simulink model "Nanogrid"  (R2026a)
settings: Solver=VariableStepAuto  StopTime=3
PreLoadFcn:
  | NanogridParam
undefined symbols (not defined in the file): baseLoad, bessSystem, bessVoltage, DiscIntNeverNeededParam, ee_sli_rtmsupport, gcbh, gflInverter, gfmInverter, nanoLoad, PV, PVInverter, ref, solar, solarInsolationChange, Ts
libraries: nesl_utility x51, eeGeneralControl x38, ee_lib x33, fl_lib x24, simulink x20, eeTransforms x13, slpidlib x8, nesl_utility_internal x4, sl_signal_attributes x4, sl_discontinuities x4, eeSinusoidalMeasurementV2 x3, batteryecm_lib x2
(part 2 of 6)

== system Nanogrid/BESS Integrated/Detailed/BESS Controller ==
  VRef : Inport
  FRef : Inport  Port=2
  PRef : Inport  Port=3
  QRef : Inport  Port=4
  Mode : Inport  Port=5
  Reset : Inport  Port=6
  VIBus : Inport  Port=7
  Grid Following : Subsystem  VariantControl=Grid Following  mask(Grid Following Controller){mp=gflInverter.activeDroop, mv=gflInverter.reactiveDroop, P=Real power, MVA=gflInverter.ratedPower, frequency=frequency, zbase=gflInverter.baseImpedance, L=filterInductance%gflInverter.filterInductance, Imax=gflInverter.iMaxPU, Td=gflInverter.sensorDelay, Kpic=gflInverter.kpId, Kiic=gflInverter.kiId, Kd=0}
      mask prompts: mp "Real power droop cofficient"; mv "Reactive power droop cofficient"; P "Priority mode"; MVA "Base Power (V*A)"; frequency "Frequency (Hz)"; zbase "Base Impedance (Ohm)"; L "Filter Inductance (H)"; Imax "Inverter current limit (pu)"; Td "Sensor time delay (s)"; Kpic "Proportional gain"; Kiic "Integral gain"; Kd "Derevative gain"
      mask help: This block implements a Grid Following control strategy where the BESS synchronizes with an existing grid voltage and frequency. Ideal for systems where the grid is strong and the BESS acts as a power source following grid conditions.
      settings: CopyFcn=set_param(gcb,'LinkStatus','none');
      mask TypeOptions P: Real power  | Reactive power
      mask DialogControl Container4 Prompt: General
      mask DialogControl Container5 Prompt: Current Controller
      mask Display: image('gridfollowing2_2_9_7_2_1_1.png');
  Grid Forming : Subsystem  VariantControl=Grid Forming  mask(Grid Forming Controller){power=plantRating*1000, girdLineVoltage=Vac, powerFreq=frequency, dcBusVoltage=bessVoltage, measSampleTime=gfmInverter.measurementSampleTime, powerControl=Virtual Synchronous Machine, activePowerSampleTime=gfmInverter.droopControl.sampleTime, droopSlope=gfmInverter.droopControl.freqSlopeMp*350, droopT1=gfmInverter.droopControl.T1, droopT2=gfmInverter.droopControl.T2, droopTC=gfmInverter.droopControl.lpfTimeConst, vsmPmeasFilterTC=gfmInverter.vsm.PmeasTimeConst, vsmFreqDroop=gfmInverter.vsm.freqDroop, vsmInertiaTC=gfmInverter.vsm.inertiaConstant, vsmDampingConst=gfmInverter.vsm.dampingCoefficent, dampingPowerMaxLimit=gfmInverter.vsm.maxDampingPower, dampingPowerMinLimit=gfmInverter.vsm.minDampingPower, freqMeasTimeConst=gfmInverter.freqMeasTimeConst, freqOption=Constant Frequency Reference, voltreference=gfmInverter.Qcontrol.voltageReference, QVoltFilterTC=gfmInverter.Qcontrol.QmeasTimeConst, QVoltDroop=gfmInverter.Qcontrol.voltageDroop, currentLimit=Current Limiting, maxSatCurrentLimit=1%gfmInverter.currentLimit.maxSaturationCurrent, maxVICurrentLimit=gfmInverter.currentLimit.viCurrentLimit, ctLimitVirtualImp=gfmInverter.currentLimit.virImpResistanceCoeff, ctLimitXbyR=gfmInverter.currentLimit.virImpXbyR, ctLimitDelayTime=gfmInverter.currentLimit.maxSaturationDelay, currentSatTime=gfmInverter.currentLimit.satCurrentRunTime, currentVITimeConst=gfmInverter.currentLimit.viFilterTimeConst, voltControlTs=gfmInverter.controller.VoltageControlSampleTime, vdPGain=gfmInverter.controller.voltControllerKp, VdIGain=gfmInverter.controller.voltControllerKi, VdMaxCt=gfmInverter.controller.voltageMaxId, VdMinCt=gfmInverter.controller.voltageMinId, VqPGain=gfmInverter.controller.voltControllerKp, VqIGain=gfmInverter.controller.voltControllerKi, VqMaxCt=gfmInverter.controller.voltageMaxIq, VqMinCt=gfmInverter.controller.voltageMinIq, vdvqLPFTimeConst=gfmInverter.controller.voltMeasTimeConst, currentControlTs=gfmInverter.controller.CurrentControlSampleTime, filterInductance=gfmInverter.L, IdPGain=gfmInverter.controller.ctControllerKp, IdIGain=gfmInverter.controller.ctControllerKi, IqPGain=gfmInverter.controller.ctControllerKp, IqIGain=gfmInverter.controller.ctControllerKi}
      mask prompts: power "Grid forming converter power (VA)"; girdLineVoltage "Grid line voltage (V)"; powerFreq "Grid frequency (Hz)"; dcBusVoltage "DC bus voltage"; measSampleTime "Measurement sample time"; powerControl "Active Power Control"; activePowerSampleTime "Sample time (s)"; droopSlope "Power droop slope (pu, Hz/W)"; droopT1 "Lead-Lag numerator time constant (s)"; droopT2 "Lead-Lag denominator time constant (s)"; droopTC "Filter cut-off time constant (s)"; vsmPmeasFilterTC "Power measurement filter time constant (s)"; vsmFreqDroop "Frequency droop (pu,  W/Hz)"; vsmInertiaTC "Inertia constant M (pu)"; vsmDampingConst "Damping constant (pu/Hz)"; dampingPowerMaxLimit "Damping power maximum limit (pu)"; dampingPowerMinLimit "Damping power minimum limit (pu)"; freqMeasTimeConst "Frequency measurement time constant (s)"; freqOption "Damping power fequency option"; voltreference "Voltage reference value (pu)"; QVoltFilterTC "Power measurement filter time constant (s)"; QVoltDroop "Voltage droop (pu, V/VAR)"; currentLimit "Current limiting method"; maxSatCurrentLimit "Maximum current saturation (pu)"; maxVICurrentLimit "Maximum virtual impedance current (pu)"; ctLimitVirtualImp "Virtual impedance coefficient (pu.Ohm/pu.A)"; ctLimitXbyR "Virtual X/R ratio"; ctLimitDelayTime "Maximum current delay time (s)"; currentSatTime "Current limiting run time (s)"; currentVITimeConst "Filter time constant (s)"; voltControlTs "Controller sample time (s)"; vdPGain "Vd proportional gain"; VdIGain "Vd integral gain"; VdMaxCt "Vd maximum current limit (A)"; VdMinCt "Vd minimum current limit (A)"; VqPGain "Vq proportional gain"; VqIGain "Vq integral gain"; VqMaxCt "Vq maximum current limit (A)"; VqMinCt "Vq minimum current limit (A)"; vdvqLPFTimeConst "Voltage measurement filter time constant (s)"; currentControlTs "Controller sample time (s)"; filterInductance "Filter inductance (H)"; IdPGain "Id proportional gain"; IdIGain "Id integral gain"; IqPGain "Iq proportional gain"; IqIGain "Iq integral gain"
      mask help: This block implements the grid forming controller with fault ride through capability. Input to the controller are active and reactive power reference in per unit and the sensed three-phase phase current in amphere and phase voltage in volts.
      mask init:
      | powerChoice = get_param(gcb,'powerControl');
      | currentChoice = get_param(gcb,'currentLimit');
      | 
      | powerloc = [gcb, '/Power Control/ActivePowerControl']; 
      | currentloc = [gcb, '/Current Limiting/CurrentLimitingMethod'];
      | freqLoc = [gcb,'/Power Control/ActivePowerControl/vsmControl/Damping Frequency'];
      | 
      | switch powerChoice
      |     case 'Virtual Synchronous Machine'
      |         set_param(powerloc, 'LabelModeActiveChoice', 'vsm');
      |         dampingFreqChoice = get_param(gcb,'freqOption');
      |         if strcmp(dampingFreqChoice,'Use Grid Frequency Measurement')
      |             set_param(freqLoc, 'LabelModeActiveChoice', 'freqMeas');
      |         else
      |             set_param(freqLoc, 'LabelModeActiveChoice', 'constFreq');
      |         end
      |     case 'Droop Control'
      |          set_param(powerloc, 'LabelModeActiveChoice', 'droop');
      |    otherwise
      |         disp('Choose proper active power control method')
      | end
      | switch currentChoice
      |     case 'Virtual Impedance'
      |           set_param(currentloc, 'LabelModeActiveChoice', 'virimp');
      |     case 'Current Limiting'
      |          set_param(currentloc, 'LabelModeActiveChoice', 'ctSat');
      |     case 'Combining Virtual Impedance and Current Limiting'
      |             set_param(currentloc, 'LabelModeActiveChoice', 'both');
      |     otherwise
      |         disp('Choose proper current limiting method')
      | end
      settings: CopyFcn=set_param(gcb,'LinkStatus','none');
      mask TypeOptions powerControl: Virtual Synchronous Machine | Droop Control
      mask Callback powerControl:
      | h = Simulink.Mask.get(gcb);
      | slectedActivePowerControl=get_param(gcb,'powerControl');
      | %slectedActivePowerControl = h.Parameters(find(string({h.Parameters.Name}) == 'powerControl')).Value;
      | switch slectedActivePowerControl
      |     case 'Virtual Synchronous Machine'
      |         h.Parameters(find(string({h.Parameters.Name}) == 'droopSlope')).Visible = 'off';
      |         h.Parameters(find(string({h.Parameters.Name}) == 'droopTC')).Visible = 'off';
      |         h.Parameters(find(string({h.Parameters.Name}) == 'droopT1')).Visible = 'off';
      |         h.Parameters(find(string({h.Parameters.Name}) == 'droopT2')).Visible = 'off';
      |         h.Parameters(find(string({h.Parameters.Name}) == 'vsmPmeasFilterTC')).Visible = 'on';
      |         h.Parameters(find(string({h.Parameters.Name}) == 'vsmFreqDroop')).Visible = 'on';
      |         h.Parameters(find(string({h.Parameters.Name}) == 'vsmInertiaTC')).Visible = 'on';
      |         h.Parameters(find(string({h.Parameters.Name}) == 'vsmDampingConst')).Visible = 'on';
      |         h.Parameters(find(string({h.Parameters.Name}) == 'dampingPowerMaxLimit')).Visible = 'on';
      |         h.Parameters(find(string({h.Parameters.Name}) == 'dampingPowerMinLimit')).Visible = 'on';
      |         h.Parameters(find(string({h.Parameters.Name}) == 'freqOption')).Visible = 'on';
      |         h.Parameters(find(string({h.Parameters.Name}) == 'freqMeasTimeConst')).Visible = 'on';
      |     case 'Droop Control'
      |         h.Parameters(find(string({h.Parameters.Name}) == 'droopSlope')).Visible = 'on';
      |         h.Parameters(find(string({h.Parameters.Name}) == 'droopTC')).Visible = 'on';
      |         h.Parameters(find(string({h.Parameters.Name}) == 'droopT1')).Visible = 'on';
      |         h.Parameters(find(string({h.Parameters.Name}) == 'droopT2')).Visible = 'on';
      |         h.Parameters(find(string({h.Parameters.Name}) == 'vsmPmeasFilterTC')).Visible = 'off';
      |         h.Parameters(find(string({h.Parameters.Name}) == 'vsmFreqDroop')).Visible = 'off';
      |         h.Parameters(find(string({h.Parameters.Name}) == 'vsmInertiaTC')).Visible = 'off';
      |         h.Parameters(find(string({h.Parameters.Name}) == 'vsmDampingConst')).Visible = 'off';
      |         h.Parameters(find(string({h.Parameters.Name}) == 'dampingPowerMaxLimit')).Visible = 'off';
      |         h.Parameters(find(string({h.Parameters.Name}) == 'dampingPowerMinLimit')).Visible = 'off';
      |         h.Parameters(find(string({h.Parameters.Name}) == 'freqOption')).Visible = 'off';
      |         h.Parameters(find(string({h.Parameters.Name}) == 'freqMeasTimeConst')).Visible = 'on';
      | 
      |     otherwise
      |         disp('Choose proper active power control method')
      | end
      mask TypeOptions freqOption: Use Grid Frequency Measurement | Constant Frequency Reference
      mask TypeOptions currentLimit: Virtual Impedance | Current Limiting | Combining Virtual Impedance and Current Limiting
      mask Callback currentLimit:
      | currentLimit = 1;
      | h = Simulink.Mask.get(gcb);
      | currentLimitControl=get_param(gcb,'currentLimit');
      | %slectedActivePowerControl = h.Parameters(find(string({h.Parameters.Name}) == 'powerControl')).Value;
      | switch currentLimitControl
      |     case 'Virtual Impedance'
      |         h.Parameters(find(string({h.Parameters.Name}) == 'maxVICurrentLimit')).Visible = 'on';
      |         h.Parameters(find(string({h.Parameters.Name}) == 'ctLimitVirtualImp')).Visible = 'on';
      |         h.Parameters(find(string({h.Parameters.Name}) == 'ctLimitXbyR')).Visible = 'on';
      |         h.Parameters(find(string({h.Parameters.Name}) == 'maxSatCurrentLimit')).Visible = 'off';
      |         h.Parameters(find(string({h.Parameters.Name}) == 'ctLimitDelayTime')).Visible = 'off';
      |         h.Parameters(find(string({h.Parameters.Name}) == 'currentSatTime')).Visible = 'off';
      |         h.Parameters(find(string({h.Parameters.Name}) == 'currentVITimeConst')).Visible = 'on';
      | 
      | 
      |     case 'Current Limiting'
      |         h.Parameters(find(string({h.Parameters.Name}) == 'maxVICurrentLimit')).Visible = 'off';
      |         h.Parameters(find(string({h.Parameters.Name}) == 'ctLimitVirtualImp')).Visible = 'off';
      |         h.Parameters(find(string({h.Parameters.Name}) == 'ctLimitXbyR')).Visible = 'off';
      |         h.Parameters(find(string({h.Parameters.Name}) == 'maxSatCurrentLimit')).Visible = 'on';
      |         h.Parameters(find(string({h.Parameters.Name}) == 'ctLimitDelayTime')).Visible = 'on';
      |         h.Parameters(find(string({h.Parameters.Name}) == 'currentSatTime')).Visible = 'off';
      |         h.Parameters(find(string({h.Parameters.Name}) == 'currentVITimeConst')).Visible = 'off';
      | 
      |     case 'Combining Virtual Impedance and Current Limiting'
      |         h.Parameters(find(string({h.Parameters.Name}) == 'maxVICurrentLimit')).Visible = 'on';
      |         h.Parameters(find(string({h.Parameters.Name}) == 'ctLimitVirtualImp')).Visible = 'on';
      |         h.Parameters(find(string({h.Parameters.Name}) == 'ctLimitXbyR')).Visible = 'on';
      |         h.Parameters(find(string({h.Parameters.Name}) == 'maxSatCurrentLimit')).Visible = 'on';
      |         h.Parameters(find(string({h.Parameters.Name}) == 'ctLimitDelayTime')).Visible = 'off';
      |         h.Parameters(find(string({h.Parameters.Name}) == 'currentSatTime')).Visible = 'on';
      |         h.Parameters(find(string({h.Parameters.Name}) == 'currentVITimeConst')).Visible = 'on';
      | 
      |     otherwise
      |         disp('Choose proper current limiting method')
      | end
      mask DialogControl ParameterGroupVar Prompt: Grid Forming Control Parameters
      mask DialogControl Container8 Prompt: Grid-forming Converter Specification
      mask DialogControl Pcontrolgrp Prompt: Active Power Controller Parameters
      mask DialogControl QcontrolGrp Prompt: Reactive Power Controller Parameters
      mask DialogControl faultRideThroughGrp Prompt: Fault Ride Through Parameters
      mask DialogControl voltControlgrp Prompt: Voltage Controller Parameters
      mask DialogControl Container15currentContGrp Prompt: Current Controller Parameters
      mask Display: image('gfmGridFormingConverterVSM1_1_7_7_2.png');
  mabc : Outport

== system Nanogrid/BESS Integrated/Detailed/BESS Plant ==
  mabc : Inport
  Battery : batteryecm_lib/Battery  Vnom=bessVoltage V  prm_dir=simscape.enum.battery.prm_dir.disabled  R1_dis=2 Ohm  R1_ch=2 Ohm  R1=0.001 Ohm  prm_AH=simscape.enum.battery.prm_AH.finite  AH=bessSystem.capacityAh A*hr  V1=0.95*bessVoltage V  AH1=0.5*bessSystem.capacityAh A*hr  prm_R2=simscape.enum.battery.prm_R2.disabled  R2=2000 Ohm  Tmeas=298.15 K  charge_measurement_port=simscape.enum.battery.enable.yes  prm_dyn=simscape.enum.battery.prm_dyn.off  Rp1=0.005 Ohm  tau1=30 s  Rp2=0.005 Ohm  tau2=30 s  Rp3=0.005 Ohm  tau3=30 s  Rp4=0.005 Ohm  tau4=30 s  Rp5=0.005 Ohm  tau5=30 s  prm_fade=simscape.enum.battery.prm_fade.disabled  N_fade=100  AH_fade=45 A*hr  R1_fade=2.02 Ohm  R1_ch_fade=2.02 Ohm  V1_fade=10.35 V  prm_age=simscape.enum.battery.prm_age.disabled  prm_age_OCV=simscape.enum.battery.prm_age_OCV.OCV  OCV_age=0.9  SOC_age=60  Tmeas_age=298.15 K  delta_time_age_vec=[0] d  temperature_age_vec=[273] K  OCV_scaling_age=2.2134e6  OCV_offset_age=1.632e6  temp_exp_age=0.515833569 V  t_exp_age=0.75  Vnom_T2=12 V  R1_T2=2.2 Ohm  R1_T2_dis=2.2 Ohm  R1_T2_ch=2.2 Ohm  V1_T2=11.4 V  R2_T2=2200 Ohm  Rp1_T2=0.005 Ohm  tau1_T2=30 s  Rp2_T2=0.005 Ohm  tau2_T2=30 s  Rp3_T2=0.005 Ohm  tau3_T2=30 s  Rp4_T2=0.005 Ohm  tau4_T2=30 s  Rp5_T2=0.005 Ohm  tau5_T2=30 s  Tmeas2=273.15 K  thermal_port=simscape.enum.thermaleffects.omit  thermal_mass=30000 J/K  i_specify=off  i_priority=None  i=0 A  i_nominal_specify=off  i_nominal_value=1  i_nominal_unit=A  v_specify=off  v_priority=None  v=0 V  v_nominal_specify=off  v_nominal_value=1  v_nominal_unit=V  charge_specify=on  charge_priority=High  charge=bessSystem.initialSOC*bessSystem.capacityAh A*hr  charge_nominal_specify=off  charge_nominal_value=1  charge_nominal_unit=A*hr  num_cycles_specify=off  num_cycles_priority=High  num_cycles=0  num_cycles_nominal_specify=off  num_cycles_nominal_value=1  num_cycles_nominal_unit=1  temperature_specify=off  temperature_priority=High  temperature=298.15 K  temperature_nominal_specify=off  temperature_nominal_value=1  temperature_nominal_unit=K
  Converter : Subsystem  InitFcn=%solar.mask.restoreConverterLink(gcb);  Variant=on  VariantControlMode=label  LabelModeActiveChoice=Average  mask{converterFidelity=Average, fSw=fSw}
      mask prompts: converterFidelity "Converter Fidelity"; fSw "Switching Frequency (kHz)"
      settings: PreSaveFcn=%solar.mask.restoreConverterLink  CloseFcn=%solar.mask.restoreConverterLink
      mask TypeOptions converterFidelity: Average | Switching
      mask Callback converterFidelity: component.mask.converterFidelity(gcb);
      mask DialogControl editSwitch Prompt: Edit converter parameters
      mask DialogControl editSwitch Callback:
      | converterFidelity = get_param(gcb,'converterFidelity');
      | blockPath = [gcb,'/',converterFidelity,'/','Converter'];
      | component.mask.openBlock(blockPath);
  Electrical Reference1 : fl_lib/Electrical/Electrical Elements/Electrical Reference
  PS-Simulink Converter : nesl_utility/PS-Simulink Converter  PhysicalDomain=network_engine_domain  SubClassName=ps_output  LeftPortType=input  RightPortType=output  PseudoPeriodic=off  Frequencies=[]  VectorFormat=inherit  Unit=inherit  AffineConversion=off
  ~ : PMIOPort  Side=Right
  SOC : Outport
  wires:
  PS-Simulink Converter/1 -> SOC/1
  mabc/1 -> Converter/1(mabc)
  connections:
  PS-Simulink Converter/LConn1 -- Battery/LConn2
  ~/RConn1 -- Converter/RConn1
  Battery/LConn1 -- Converter/LConn1
  Converter/LConn2 -- Electrical Reference1/LConn1 -- Battery/RConn1

== system Nanogrid/BESS Integrated/Detailed/Filter & Measurements ==
  SOC : Inport
  Current and Voltage Sensor (Three-Phase) : ee_lib/Sensors & Transducers/Current and Voltage Sensor (Three-Phase)  port_option=ee.enum.threePhasePort.composite  vMeasurementType=ee.enum.vmeasurement.lg  outputUnit=ee.enum.unit.pu  SRated=plantRating*1000 A*V  VRated=Vac V  I_specify=off  I_priority=None  I=[ 0 0 0 ] A  I_nominal_specify=off  I_nominal_value=1  I_nominal_unit=A  V_specify=off  V_priority=None  V=[ 0 0 0 ] V  V_nominal_specify=off  V_nominal_value=1  V_nominal_unit=V
  Gain : Gain  Gain=1/(plantRating*1000)
  Gain1 : Gain  Gain=1/(plantRating*1000)
  Low-Pass Filter (Discrete or Continuous) : eeGeneralControl/Low-Pass Filter (Discrete or Continuous)  K=1  T=0.02  B=inf  A=-inf  init_option=Inherited from block input  x0=0  Ts=Ts
  Low-Pass Filter (Discrete or Continuous)1 : eeGeneralControl/Low-Pass Filter (Discrete or Continuous)  K=1  T=0.02  B=inf  A=-inf  init_option=Inherited from block input  x0=0  Ts=Ts
  PLL & Measurements : Subsystem
      mask Display: image('PLL_9_7_2.png');
  PS-Simulink Converter2 : nesl_utility_internal/PS-Simulink Converter  PhysicalDomain=network_engine_domain  SubClassName=ps_output  LeftPortType=input  RightPortType=output  PseudoPeriodic=off  Frequencies=[]  VectorFormat=1-D array  Unit=V  AffineConversion=off
  PS-Simulink Converter3 : nesl_utility_internal/PS-Simulink Converter  PhysicalDomain=network_engine_domain  SubClassName=ps_output  LeftPortType=input  RightPortType=output  PseudoPeriodic=off  Frequencies=[]  VectorFormat=1-D array  Unit=A  AffineConversion=off
  PS-Simulink Converter6 : nesl_utility_internal/PS-Simulink Converter  PhysicalDomain=network_engine_domain  SubClassName=ps_output  LeftPortType=input  RightPortType=output  PseudoPeriodic=off  Frequencies=[]  VectorFormat=1-D array  Unit=W  AffineConversion=off
  PS-Simulink Converter7 : nesl_utility_internal/PS-Simulink Converter  PhysicalDomain=network_engine_domain  SubClassName=ps_output  LeftPortType=input  RightPortType=output  PseudoPeriodic=off  Frequencies=[]  VectorFormat=1-D array  Unit=V*A  AffineConversion=off
  Power Sensor (Three-Phase)1 : ee_lib/Sensors & Transducers/Power Sensor (Three-Phase)  port_option=ee.enum.threePhasePort.composite  load_type=ee.enum.passive.type_balanced.balanced  f0=60 Hz
  RLC (Three-Phase) : ee_lib/Passive/RLC Assemblies/RLC (Three-Phase)  port_option=ee.enum.threePhasePort.composite  component_structure=ee.enum.rlc.structure.SeriesRL  R=gfmInverter.lineResistance Ohm  L=gfmInverter.L H  C=1e-6 F  R_parasitic=0 Ohm  G_parasitic=0 1/Ohm  IL_specify=on  IL_priority=None  IL=[0, 0, 0] A  IL_nominal_specify=off  IL_nominal_value=1  IL_nominal_unit=A  VC_specify=off  VC_priority=High  VC=[0, 0, 0] V  VC_nominal_specify=off  VC_nominal_value=1  VC_nominal_unit=V
  In : PMIOPort  Side=Left
  ~ : PMIOPort  Port=2  Side=Right
  VIBus : Outport
  Out Bus Element : Outport  Port=2  PortName=Meas  Element=voltage
  Out Bus Element1 : Outport  Port=2  PortName=Meas  Element=current
  Out Bus Element2 : Outport  Port=2  PortName=Meas  Element=activePower
  Out Bus Element3 : Outport  Port=2  PortName=Meas  Element=reactivePower
  BusElementOut : Outport  Port=2  PortName=Meas  Element=SOC
  wires:
  SOC/1 -> BusElementOut/1
  Gain1/1 -> Out Bus Element3/1
  Gain/1 -> Out Bus Element2/1
  PS-Simulink Converter2/1 -> Out Bus Element/1, PLL & Measurements/1(V)
  PS-Simulink Converter6/1 -> Low-Pass Filter (Discrete or Continuous)1/1
  PS-Simulink Converter7/1 -> Low-Pass Filter (Discrete or Continuous)/1
  PS-Simulink Converter3/1 -> Out Bus Element1/1, PLL & Measurements/2(I)
  Low-Pass Filter (Discrete or Continuous)/1 -> Gain1/1
  Low-Pass Filter (Discrete or Continuous)1/1 -> Gain/1
  PLL & Measurements/1(VIbus) -> VIBus/1
  connections:
  Power Sensor (Three-Phase)1/LConn1 -- Current and Voltage Sensor (Three-Phase)/RConn3
  PS-Simulink Converter2/LConn1 -- Current and Voltage Sensor (Three-Phase)/RConn1
  Current and Voltage Sensor (Three-Phase)/RConn2 -- PS-Simulink Converter3/LConn1
  Power Sensor (Three-Phase)1/LConn2 -- PS-Simulink Converter6/LConn1
  Power Sensor (Three-Phase)1/LConn3 -- PS-Simulink Converter7/LConn1
  RLC (Three-Phase)/RConn1 -- Current and Voltage Sensor (Three-Phase)/LConn1
  Power Sensor (Three-Phase)1/RConn1 -- ~/RConn1
  In/RConn1 -- RLC (Three-Phase)/LConn1

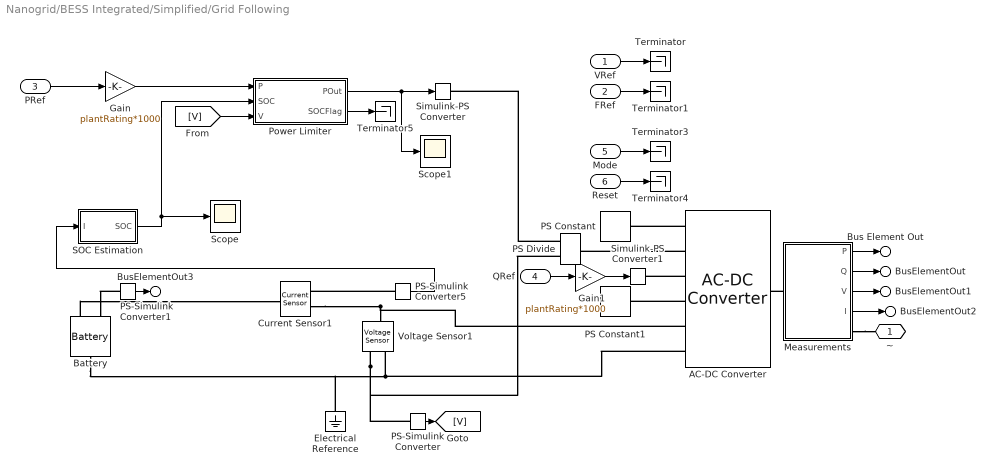
== system Nanogrid/BESS Integrated/Simplified/Grid Following ==
  VRef : Inport
  FRef : Inport  Port=2
  PRef : Inport  Port=3
  QRef : Inport  Port=4
  Mode : Inport  Port=5
  Reset : Inport  Port=6
  AC-DC Converter : custom_lib/AC-DC Converter  port_option=ee.enum.threePhasePort.composite  FRated=frequency Hz  Vline_rms_ini=Vac/4 V  VRated=Vac V  Vang_ini=0 deg  IMaxPU=iMaxPU  PRated=plantRating kW  efficiency=efficiency
      settings: InternalSimscapePortConfiguration="{\"Bottom\":[],\"Left\":[{\"id\":\"Vref\",\"label\":\"Vref\",\"type\":\"input\"},{\"id\":\"Iref\",\"label\":\"Iref\",\"type\":\"input\"},{\"id\":\"Qref\",\"label\":\"Qref\",\"type\":\"input\"},{\"id\":\"Mode\",\"label\":\"Mode\",\"type\":\"input\"},{\"id\":\"p\",\"label\":\"+\",\"type\":\"foundation.electrical.electrical\"},{\"id\":\"n\",\"label\":\"-\",\"type\":\"foundation.electrical.electrical\"}],\"Right\":[{\"id\":\"N\",\"label\":\"~\",\"type\":\"foundation.electrical.three_phase\"}],\"Top\":[]}"
  Battery : batteryecm_lib/Battery  Vnom=bessVoltage V  prm_dir=simscape.enum.battery.prm_dir.disabled  R1_dis=2 Ohm  R1_ch=2 Ohm  R1=1e-3 Ohm  prm_AH=simscape.enum.battery.prm_AH.infinite  AH=50 A*hr  V1=11.5 V  AH1=25 A*hr  prm_R2=simscape.enum.battery.prm_R2.disabled  R2=2000 Ohm  Tmeas=298.15 K  charge_measurement_port=simscape.enum.battery.enable.yes  prm_dyn=simscape.enum.battery.prm_dyn.off  Rp1=0.005 Ohm  tau1=30 s  Rp2=0.005 Ohm  tau2=30 s  Rp3=0.005 Ohm  tau3=30 s  Rp4=0.005 Ohm  tau4=30 s  Rp5=0.005 Ohm  tau5=30 s  prm_fade=simscape.enum.battery.prm_fade.disabled  N_fade=100  AH_fade=45 A*hr  R1_fade=2.02 Ohm  R1_ch_fade=2.02 Ohm  V1_fade=10.35 V  prm_age=simscape.enum.battery.prm_age.disabled  prm_age_OCV=simscape.enum.battery.prm_age_OCV.OCV  OCV_age=0.9  SOC_age=60  Tmeas_age=298.15 K  delta_time_age_vec=[0] d  temperature_age_vec=[273] K  OCV_scaling_age=2.2134e6  OCV_offset_age=1.632e6  temp_exp_age=0.515833569 V  t_exp_age=0.75  Vnom_T2=12 V  R1_T2=2.2 Ohm  R1_T2_dis=2.2 Ohm  R1_T2_ch=2.2 Ohm  V1_T2=11.4 V  R2_T2=2200 Ohm  Rp1_T2=0.005 Ohm  tau1_T2=30 s  Rp2_T2=0.005 Ohm  tau2_T2=30 s  Rp3_T2=0.005 Ohm  tau3_T2=30 s  Rp4_T2=0.005 Ohm  tau4_T2=30 s  Rp5_T2=0.005 Ohm  tau5_T2=30 s  Tmeas2=273.15 K  thermal_port=simscape.enum.thermaleffects.omit  thermal_mass=30000 J/K  i_specify=off  i_priority=None  i=0 A  i_nominal_specify=off  i_nominal_value=1  i_nominal_unit=A  v_specify=off  v_priority=None  v=0 V  v_nominal_specify=off  v_nominal_value=1  v_nominal_unit=V  charge_specify=off  charge_priority=High  charge=50 A*hr  charge_nominal_specify=off  charge_nominal_value=1  charge_nominal_unit=A*hr  num_cycles_specify=off  num_cycles_priority=High  num_cycles=0  num_cycles_nominal_specify=off  num_cycles_nominal_value=1  num_cycles_nominal_unit=1  temperature_specify=off  temperature_priority=High  temperature=298.15 K  temperature_nominal_specify=off  temperature_nominal_value=1  temperature_nominal_unit=K
      settings: InternalSimscapePortConfiguration="{\"Bottom\":[],\"Left\":[{\"id\":\"p\",\"label\":\"+\",\"type\":\"foundation.electrical.electrical\"},{\"id\":\"q\",\"label\":\"q\",\"type\":\"output\"}],\"Right\":[{\"id\":\"n\",\"label\":\"-\",\"type\":\"foundation.electrical.electrical\"}],\"Top\":[]}"
  Current Sensor1 : fl_lib/Electrical/Electrical Sensors/Current Sensor
  Electrical Reference : fl_lib/Electrical/Electrical Elements/Electrical Reference
  Gain : Gain  Gain=plantRating*1000
  Gain1 : Gain  Gain=plantRating*1000
  Measurements : Subsystem
  PS Constant : fl_lib/Physical Signals/Sources/PS Constant  constant=0
  PS Constant1 : fl_lib/Physical Signals/Sources/PS Constant  constant=1
  PS Divide : fl_lib/Physical Signals/Functions/PS Divide
  PS-Simulink Converter : nesl_utility/PS-Simulink Converter  PhysicalDomain=network_engine_domain  SubClassName=ps_output  LeftPortType=input  RightPortType=output  PseudoPeriodic=off  Frequencies=[]  VectorFormat=inherit  Unit=inherit  AffineConversion=off
  PS-Simulink Converter1 : nesl_utility/PS-Simulink Converter  PhysicalDomain=network_engine_domain  SubClassName=ps_output  LeftPortType=input  RightPortType=output  PseudoPeriodic=off  Frequencies=[]  VectorFormat=inherit  Unit=inherit  AffineConversion=off
  PS-Simulink Converter5 : nesl_utility/PS-Simulink Converter  PhysicalDomain=network_engine_domain  SubClassName=ps_output  LeftPortType=input  RightPortType=output  PseudoPeriodic=off  Frequencies=[]  VectorFormat=inherit  Unit=inherit  AffineConversion=off
  Power Limiter : Subsystem
  SOC Estimation : Subsystem
  Scope : Scope
      settings: ActiveDisplayYMinimum=-1  ActiveDisplayYMaximum=1  DataLoggingVariableName=ScopeData21
  Scope1 : Scope
  Simulink-PS Converter : nesl_utility/Simulink-PS Converter  PhysicalDomain=network_engine_domain  SubClassName=ps_input  LeftPortType=input  RightPortType=output  PseudoPeriodic=off  Frequencies=[]  NoiseDistribution=none  NoiseParameters=[]  Unit=V*A  AffineConversion=off  FilteringAndDerivatives=provide  SimscapeFilterOrder=1  InputFilterTimeConstant=0.001  UdotUserProvided=0
  Simulink-PS Converter1 : nesl_utility/Simulink-PS Converter  PhysicalDomain=network_engine_domain  SubClassName=ps_input  LeftPortType=input  RightPortType=output  PseudoPeriodic=off  Frequencies=[]  NoiseDistribution=none  NoiseParameters=[]  Unit=1  AffineConversion=off  FilteringAndDerivatives=provide  SimscapeFilterOrder=1  InputFilterTimeConstant=0.001  UdotUserProvided=0
  Terminator{,1,3..5} (5 alike) : Terminator
  Voltage Sensor1 : fl_lib/Electrical/Electrical Sensors/Voltage Sensor
  ~ : PMIOPort  Side=Right
  Bus Element Out : Outport  PortName=Meas  Element=activePower
  BusElementOut : Outport  PortName=Meas  Element=reactivePower
  BusElementOut1 : Outport  PortName=Meas  Element=voltage
  BusElementOut2 : Outport  PortName=Meas  Element=current
  BusElementOut3 : Outport  PortName=Meas  Element=SOC
  wires:
  PS-Simulink Converter1/1 -> BusElementOut3/1
  Measurements/4(I) -> BusElementOut2/1
  Measurements/2(Q) -> BusElementOut/1
  Measurements/3(V) -> BusElementOut1/1
  Measurements/1(P) -> Bus Element Out/1
  Gain1/1 -> Simulink-PS Converter1/1
  PRef/1 -> Gain/1
  Power Limiter/2(SOCFlag) -> Terminator5/1
  Power Limiter/1(POut) -> Scope1/1, Simulink-PS Converter/1
  Reset/1 -> Terminator4/1
  SOC Estimation/1(SOC) -> Scope/1, Power Limiter/2(SOC)
  [V] -> Power Limiter/3(V)
  Mode/1 -> Terminator3/1
  PS-Simulink Converter5/1 -> SOC Estimation/1(I)
  QRef/1 -> Gain1/1
  FRef/1 -> Terminator1/1
  VRef/1 -> Terminator/1
  PS-Simulink Converter/1 -> [V]
  Gain/1 -> Power Limiter/1(P)
  connections:
  PS-Simulink Converter1/LConn1 -- Battery/LConn2
  Measurements/RConn1 -- ~/RConn1
  Measurements/LConn1 -- AC-DC Converter/RConn1
  AC-DC Converter/LConn3 -- Simulink-PS Converter1/RConn1
  AC-DC Converter/LConn1 -- PS Constant/RConn1
  Battery/LConn1 -- Current Sensor1/LConn1
  PS Divide/LConn1 -- Simulink-PS Converter/RConn1
  PS-Simulink Converter5/LConn1 -- Current Sensor1/RConn1
  AC-DC Converter/LConn2 -- PS Divide/RConn1
  AC-DC Converter/LConn4 -- PS Constant1/RConn1
  AC-DC Converter/LConn5 -- Voltage Sensor1/LConn1 -- Current Sensor1/RConn2
  AC-DC Converter/LConn6 -- Voltage Sensor1/RConn2 -- Electrical Reference/LConn1 -- Battery/RConn1
  Voltage Sensor1/RConn1 -- PS-Simulink Converter/LConn1 -- PS Divide/LConn2

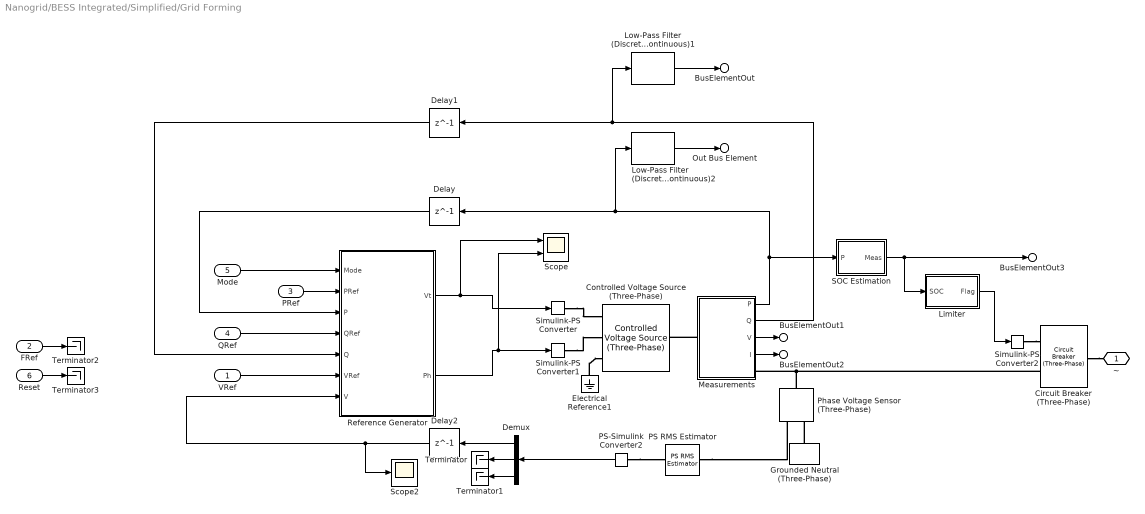
== system Nanogrid/BESS Integrated/Simplified/Grid Forming ==
  VRef : Inport
  FRef : Inport  Port=2
  PRef : Inport  Port=3
  QRef : Inport  Port=4
  Mode : Inport  Port=5
  Reset : Inport  Port=6
  Circuit Breaker (Three-Phase) : ee_lib/Switches & Breakers/Circuit Breaker (Three-Phase)  R_closed=0.001 Ohm  G_open=1e-6 1/Ohm  threshold=0.5 V  breaker_behavior=ee.enum.switches.breakerBehavior.zeroCrossingDisable
      settings: InternalSimscapePortConfiguration="{\"Bottom\":[],\"Left\":[{\"id\":\"vT\",\"label\":\"vT\",\"type\":\"input\"},{\"id\":\"N1\",\"label\":\"~1\",\"type\":\"foundation.electrical.three_phase\"}],\"Right\":[{\"id\":\"N2\",\"label\":\"~2\",\"type\":\"foundation.electrical.three_phase\"}],\"Top\":[]}"
  Controlled Voltage Source (Three-Phase) : ee_lib/Sources/Controlled Voltage Source (Three-Phase)  input_option=ee.enum.inputType.singleFreqAC  FRated=frequency Hz
      settings: InternalSimscapePortConfiguration="{\"Bottom\":[],\"Left\":[{\"id\":\"Vt\",\"label\":\"Vt\",\"type\":\"input\"},{\"id\":\"ph\",\"label\":\"ph\",\"type\":\"input\"},{\"id\":\"n\",\"label\":\"n\",\"type\":\"foundation.electrical.electrical\"}],\"Right\":[{\"id\":\"N\",\"label\":\"~\",\"type\":\"foundation.electrical.three_phase\"}],\"Top\":[]}"
  Delay : Delay  DelayLength=1
  Delay1 : Delay  DelayLength=1
  Delay2 : Delay  DelayLength=1
  Demux : Demux  Outputs=3
  Electrical Reference1 : fl_lib/Electrical/Electrical Elements/Electrical Reference
  Grounded Neutral (Three-Phase) : ee_lib/Connectors & References/Grounded Neutral (Three-Phase)
  Limiter : Subsystem
  Low-Pass Filter (Discrete or Continuous)1 : eeGeneralControl/Low-Pass Filter (Discrete or Continuous)  K=1  T=0.1  B=inf  A=-inf  init_option=Inherited from block input  x0=0  Ts=-1
  Low-Pass Filter (Discrete or Continuous)2 : eeGeneralControl/Low-Pass Filter (Discrete or Continuous)  K=1  T=0.1  B=inf  A=-inf  init_option=Inherited from block input  x0=0  Ts=-1
  Measurements : Subsystem
  PS RMS Estimator : fl_lib/Physical Signals/Periodic Operators/PS RMS Estimator  f0=frequency Hz
      settings: InternalSimscapePortConfiguration="{\"Bottom\":[],\"Left\":[{\"id\":\"I\",\"label\":\"\",\"type\":\"input\"}],\"Right\":[{\"id\":\"O\",\"label\":\"\",\"type\":\"output\"}],\"Top\":[]}"
  PS-Simulink Converter2 : nesl_utility/PS-Simulink Converter  PhysicalDomain=network_engine_domain  SubClassName=ps_output  LeftPortType=input  RightPortType=output  PseudoPeriodic=off  Frequencies=[]  VectorFormat=inherit  Unit=inherit  AffineConversion=off
  Phase Voltage Sensor (Three-Phase) : ee_lib/Sensors & Transducers/Phase Voltage Sensor (Three-Phase)
  Reference Generator : Subsystem  mask{activeDroop=activeDroop, reactiveDroop=reactiveDroop, systemVoltage=Vac, systemFrequency=frequency, basePower=plantRating*1000}
      mask prompts: activeDroop "Active Droop"; reactiveDroop "Reactive Droop"; systemVoltage "AC Voltage"; systemFrequency "Frequency"; basePower "Base Power"
  SOC Estimation : Subsystem
  Scope : Scope  NumInputPorts=2
      settings: ActiveDisplayYMinimum=603.75  ActiveDisplayYMaximum=776.25000000000011
  Scope2 : Scope
  Simulink-PS Converter : nesl_utility/Simulink-PS Converter  PhysicalDomain=network_engine_domain  SubClassName=ps_input  LeftPortType=input  RightPortType=output  PseudoPeriodic=off  Frequencies=[]  NoiseDistribution=none  NoiseParameters=[]  Unit=1  AffineConversion=off  FilteringAndDerivatives=provide  SimscapeFilterOrder=1  InputFilterTimeConstant=0.001  UdotUserProvided=0
  Simulink-PS Converter1 : nesl_utility/Simulink-PS Converter  PhysicalDomain=network_engine_domain  SubClassName=ps_input  LeftPortType=input  RightPortType=output  PseudoPeriodic=off  Frequencies=[]  NoiseDistribution=none  NoiseParameters=[]  Unit=1  AffineConversion=off  FilteringAndDerivatives=provide  SimscapeFilterOrder=1  InputFilterTimeConstant=0.001  UdotUserProvided=0
  Simulink-PS Converter2 : nesl_utility/Simulink-PS Converter  PhysicalDomain=network_engine_domain  SubClassName=ps_input  LeftPortType=input  RightPortType=output  PseudoPeriodic=off  Frequencies=[]  NoiseDistribution=none  NoiseParameters=[]  Unit=1  AffineConversion=off  FilteringAndDerivatives=provide  SimscapeFilterOrder=1  InputFilterTimeConstant=0.001  UdotUserProvided=0
  Terminator{,1..3} (4 alike) : Terminator
  ~ : PMIOPort  Side=Right
  Out Bus Element : Outport  PortName=Meas  Element=activePower
  BusElementOut : Outport  PortName=Meas  Element=reactivePower
  BusElementOut1 : Outport  PortName=Meas  Element=voltage
  BusElementOut2 : Outport  PortName=Meas  Element=current
  BusElementOut3 : Outport  PortName=Meas  Element=SOC
  wires:
  Limiter/1(Flag) -> Simulink-PS Converter2/1
  PRef/1 -> Reference Generator/2(PRef)
  Low-Pass Filter (Discrete or Continuous)2/1 -> Out Bus Element/1
  Low-Pass Filter (Discrete or Continuous)1/1 -> BusElementOut/1
  Mode/1 -> Reference Generator/1(Mode)
  Delay1/1 -> Reference Generator/5(Q)
  FRef/1 -> Terminator2/1
  Reference Generator/1(Vt) -> Scope/1, Simulink-PS Converter/1
  VRef/1 -> Reference Generator/6(VRef)
  QRef/1 -> Reference Generator/4(QRef)
  Demux/1 -> Delay2/1
  Delay/1 -> Reference Generator/3(P)
  PS-Simulink Converter2/1 -> Demux/1
  Reference Generator/2(Ph) -> Scope/2, Simulink-PS Converter1/1
  Demux/2 -> Terminator/1
  Delay2/1 -> Reference Generator/7(V), Scope2/1
  Reset/1 -> Terminator3/1
  Demux/3 -> Terminator1/1
  Measurements/1(P) -> SOC Estimation/1(P), Low-Pass Filter (Discrete or Continuous)2/1, Delay/1
  Measurements/2(Q) -> Low-Pass Filter (Discrete or Continuous)1/1, Delay1/1
  Measurements/3(V) -> BusElementOut1/1
  Measurements/4(I) -> BusElementOut2/1
  SOC Estimation/1(Meas) -> Limiter/1(SOC), BusElementOut3/1
  connections:
  Simulink-PS Converter2/RConn1 -- Circuit Breaker (Three-Phase)/LConn1
  Circuit Breaker (Three-Phase)/RConn1 -- ~/RConn1
  PS-Simulink Converter2/LConn1 -- PS RMS Estimator/RConn1
  Measurements/LConn1 -- Controlled Voltage Source (Three-Phase)/RConn1
  Simulink-PS Converter1/RConn1 -- Controlled Voltage Source (Three-Phase)/LConn2
  Electrical Reference1/LConn1 -- Controlled Voltage Source (Three-Phase)/LConn3
  Circuit Breaker (Three-Phase)/LConn2 -- Measurements/RConn1 -- Phase Voltage Sensor (Three-Phase)/LConn1
  PS RMS Estimator/LConn1 -- Phase Voltage Sensor (Three-Phase)/RConn1
  Simulink-PS Converter/RConn1 -- Controlled Voltage Source (Three-Phase)/LConn1
  Grounded Neutral (Three-Phase)/LConn1 -- Phase Voltage Sensor (Three-Phase)/RConn2

== system Nanogrid/Solar Plant Integrated/Detailed/Measurements ==
  Current and Voltage Sensor (Three-Phase)5 : ee_lib/Sensors & Transducers/Current and Voltage Sensor (Three-Phase)  port_option=ee.enum.threePhasePort.composite  vMeasurementType=ee.enum.vmeasurement.lg  outputUnit=ee.enum.unit.pu  SRated=plantRating*1000 A*V  VRated=Vac V  I_specify=off  I_priority=None  I=[0, 0, 0] A  I_nominal_specify=off  I_nominal_value=1  I_nominal_unit=A  V_specify=off  V_priority=None  V=[0, 0, 0] V  V_nominal_specify=off  V_nominal_value=1  V_nominal_unit=V
  Gain : Gain  Gain=1/(plantRating*1000)
  Gain1 : Gain  Gain=1/(plantRating*1000)
  Low-Pass Filter (Discrete or Continuous)1 : eeGeneralControl/Low-Pass Filter (Discrete or Continuous)  K=1  T=0.1  B=inf  A=-inf  init_option=Inherited from block input  x0=0  Ts=-1
  Low-Pass Filter (Discrete or Continuous)2 : eeGeneralControl/Low-Pass Filter (Discrete or Continuous)  K=1  T=0.1  B=inf  A=-inf  init_option=Inherited from block input  x0=0  Ts=-1
  PS-Simulink Converter{,1..3} (4 alike) : nesl_utility/PS-Simulink Converter  PhysicalDomain=network_engine_domain  SubClassName=ps_output  LeftPortType=input  RightPortType=output  PseudoPeriodic=off  Frequencies=[]  VectorFormat=inherit  Unit=inherit  AffineConversion=off
  Power Sensor (Three-Phase) : ee_lib/Sensors & Transducers/Power Sensor (Three-Phase)  port_option=ee.enum.threePhasePort.composite  load_type=ee.enum.passive.type_balanced.balanced  f0=60 Hz
  In : PMIOPort  Side=Left
  ~ : PMIOPort  Port=2  Side=Right
  P : Outport
  Q : Outport  Port=2
  V : Outport  Port=3
  I : Outport  Port=4
  wires:
  Gain1/1 -> Q/1
  Gain/1 -> P/1
  PS-Simulink Converter3/1 -> I/1
  PS-Simulink Converter2/1 -> V/1
  Low-Pass Filter (Discrete or Continuous)2/1 -> Gain1/1
  Low-Pass Filter (Discrete or Continuous)1/1 -> Gain/1
  PS-Simulink Converter1/1 -> Low-Pass Filter (Discrete or Continuous)2/1
  PS-Simulink Converter/1 -> Low-Pass Filter (Discrete or Continuous)1/1
  connections:
  PS-Simulink Converter3/LConn1 -- Current and Voltage Sensor (Three-Phase)5/RConn2
  Power Sensor (Three-Phase)/RConn1 -- Current and Voltage Sensor (Three-Phase)5/LConn1
  PS-Simulink Converter1/LConn1 -- Power Sensor (Three-Phase)/LConn3
  ~/RConn1 -- Current and Voltage Sensor (Three-Phase)5/RConn3
  In/RConn1 -- Power Sensor (Three-Phase)/LConn1
  PS-Simulink Converter/LConn1 -- Power Sensor (Three-Phase)/LConn2
  PS-Simulink Converter2/LConn1 -- Current and Voltage Sensor (Three-Phase)5/RConn1

== system Nanogrid/Solar Plant Integrated/Detailed/PV Plant & Controller ==
  note: Controller
  note: Plant
  Insolation : Inport
  Pref : Inport  Port=2
  Qref : Inport  Port=3
  Vabc : Inport  Port=4
  Iabc : Inport  Port=5
  Mode : Inport  Port=6
  Controller : Subsystem
  Delay : Delay  DelayLength=1
  PV Plant : Subsystem  InitFcn=%solar.mask.restoreSolarLink(gcb);  mask(Solar Plant){capDC=capacitance, converterFidelity=Average, fSw=fSw, ratedVoltage=Vac, nSeries=nSeries, nParallel=nParallel}
      mask prompts: capDC "DC bus capacitance (F)"; converterFidelity "Converter Fidelity"; fSw "Switching Frequency (kHz)"; ratedVoltage "Rated voltage on AC side (V)"; nSeries "Number of panels in series"; nParallel "Number of panels in parallel"
      mask help: This block represents the physical interface between the solar panels and the power converter. It models the electrical and dynamic characteristics of the solar panels connected to a converter, while expecting an external control signal for operation
      settings: CopyFcn=set_param(gcbh,'LinkStatus','none');  PreSaveFcn=%solar.mask.restoreSolarLink(gcb);  CloseFcn=%solar.mask.restoreSolarLink(gcb);
      mask TypeOptions converterFidelity: Converter/converterFidelity
      mask Callback converterFidelity: component.mask.converterFidelityPlant;
      mask TypeOptions fSw: Converter/fSw
      mask DialogControl Container4 Prompt: General
      mask DialogControl editSolarCell Prompt: Edit Solar Cell Parameters
      mask DialogControl editSolarCell Callback:
      | blockPath = [gcb,'/','PV Array'];
      | component.mask.openBlock(blockPath);;
      mask DialogControl editConverter Prompt: Edit converter parameters
      mask DialogControl editConverter Callback:
      | converterFidelity = get_param(gcb,'converterFidelity');
      | blockPath = [gcb,'/','Converter','/',converterFidelity,'/','Converter'];
      | component.mask.openBlock(blockPath);
      mask Display: image('solar1.png');
  Scope1 : Scope
      settings: ActiveDisplayYMinimum=-2.35685  ActiveDisplayYMaximum=2.29234  DataLoggingVariableName=ScopeData4
  Sensor Dynamics : Subsystem
  Simulink-PS Converter : nesl_utility/Simulink-PS Converter  PhysicalDomain=network_engine_domain  SubClassName=ps_input  LeftPortType=input  RightPortType=output  PseudoPeriodic=off  Frequencies=[]  NoiseDistribution=none  NoiseParameters=[]  Unit=1  AffineConversion=off  FilteringAndDerivatives=provide  SimscapeFilterOrder=1  InputFilterTimeConstant=0.001  UdotUserProvided=0
  abc : PMIOPort  Side=Right
  wires:
  PV Plant/2(V) -> Sensor Dynamics/2(Vin)
  PV Plant/1(I) -> Sensor Dynamics/1(Iin)
  Delay/1 -> PV Plant/1(mabc)
  Insolation/1 -> Simulink-PS Converter/1
  Controller/1(vabcRef (pu)) -> Scope1/1, Delay/1
  Sensor Dynamics/2(V) -> Controller/3(vdc (V))
  Sensor Dynamics/1(I) -> Controller/2(ipv (A))
  Qref/1 -> Controller/1(Qref)
  Pref/1 -> Controller/6(Pref)
  Vabc/1 -> Controller/4(Vabc)
  Iabc/1 -> Controller/5(Iabc)
  Mode/1 -> Controller/7(Mode)
  connections:
  abc/RConn1 -- PV Plant/RConn1
  PV Plant/LConn1 -- Simulink-PS Converter/RConn1

== system Nanogrid/Solar Plant Integrated/Simplified/Measurements ==
  Current and Voltage Sensor (Three-Phase)5 : ee_lib/Sensors & Transducers/Current and Voltage Sensor (Three-Phase)  vMeasurementType=ee.enum.vmeasurement.lg  outputUnit=ee.enum.unit.pu  SRated=plantRating*1000 A*V  VRated=Vac V  I_specify=off  I_priority=None  I=[0, 0, 0] A  I_nominal_specify=off  I_nominal_value=1  I_nominal_unit=A  V_specify=off  V_priority=None  V=[0, 0, 0] V  V_nominal_specify=off  V_nominal_value=1  V_nominal_unit=V
      settings: InternalSimscapePortConfiguration="{\"Bottom\":[],\"Left\":[{\"id\":\"N1\",\"label\":\"~1\",\"type\":\"foundation.electrical.three_phase\"}],\"Right\":[{\"id\":\"V_output\",\"label\":\"V\",\"type\":\"output\"},{\"id\":\"I_output\",\"label\":\"I\",\"type\":\"output\"},{\"id\":\"N2\",\"label\":\"~2\",\"type\":\"foundation.electrical.three_phase\"}],\"Top\":[]}"
  Gain : Gain  Gain=1/(plantRating*1000)
  Gain1 : Gain  Gain=1/(plantRating*1000)
  Low-Pass Filter (Discrete or Continuous)1 : eeGeneralControl/Low-Pass Filter (Discrete or Continuous)  K=1  T=0.1  B=inf  A=-inf  init_option=Inherited from block input  x0=0  Ts=-1
  Low-Pass Filter (Discrete or Continuous)2 : eeGeneralControl/Low-Pass Filter (Discrete or Continuous)  K=1  T=0.1  B=inf  A=-inf  init_option=Inherited from block input  x0=0  Ts=-1
  PS-Simulink Converter{,1..3} (4 alike) : nesl_utility/PS-Simulink Converter  PhysicalDomain=network_engine_domain  SubClassName=ps_output  LeftPortType=input  RightPortType=output  PseudoPeriodic=off  Frequencies=[]  VectorFormat=inherit  Unit=inherit  AffineConversion=off
  Power Sensor (Three-Phase) : ee_lib/Sensors & Transducers/Power Sensor (Three-Phase)  load_type=ee.enum.passive.type_balanced.balanced  f0=60 Hz
      settings: InternalSimscapePortConfiguration="{\"Bottom\":[],\"Left\":[{\"id\":\"N1\",\"label\":\"~1\",\"type\":\"foundation.electrical.three_phase\"}],\"Right\":[{\"id\":\"N2\",\"label\":\"~2\",\"type\":\"foundation.electrical.three_phase\"}],\"Top\":[{\"id\":\"Pm\",\"label\":\"P\",\"type\":\"output\"},{\"id\":\"Qm\",\"label\":\"Q\",\"type\":\"output\"}]}"
  In : PMIOPort  Side=Left
  ~ : PMIOPort  Port=2  Side=Right
  P : Outport
  Q : Outport  Port=2
  V : Outport  Port=3
  I : Outport  Port=4
  wires:
  Gain1/1 -> Q/1
  Gain/1 -> P/1
  PS-Simulink Converter3/1 -> I/1
  PS-Simulink Converter2/1 -> V/1
  Low-Pass Filter (Discrete or Continuous)2/1 -> Gain1/1
  Low-Pass Filter (Discrete or Continuous)1/1 -> Gain/1
  PS-Simulink Converter1/1 -> Low-Pass Filter (Discrete or Continuous)2/1
  PS-Simulink Converter/1 -> Low-Pass Filter (Discrete or Continuous)1/1
  connections:
  PS-Simulink Converter3/LConn1 -- Current and Voltage Sensor (Three-Phase)5/RConn2
  Power Sensor (Three-Phase)/RConn1 -- Current and Voltage Sensor (Three-Phase)5/LConn1
  PS-Simulink Converter1/LConn1 -- Power Sensor (Three-Phase)/LConn3
  ~/RConn1 -- Current and Voltage Sensor (Three-Phase)5/RConn3
  In/RConn1 -- Power Sensor (Three-Phase)/LConn1
  PS-Simulink Converter/LConn1 -- Power Sensor (Three-Phase)/LConn2
  PS-Simulink Converter2/LConn1 -- Current and Voltage Sensor (Three-Phase)5/RConn1

== system Nanogrid/BESS Integrated/Detailed/BESS Controller/Grid Following ==
  VRef : Inport
  FRef : Inport  Port=2
  PRef : Inport  Port=3
  QRef : Inport  Port=4
  Mode : Inport  Port=5
  Reset : Inport  Port=6
  In Bus Element3 : Inport  Port=7  PortName=VIBus  Element=Vd
  BusElementIn : Inport  Port=7  PortName=VIBus  Element=Vd
  In Bus Element2 : Inport  Port=7  PortName=VIBus  Element=Vq
  In Bus Element7 : Inport  Port=7  PortName=VIBus  Element=Theta
  BusElementIn1 : Inport  Port=7  PortName=VIBus  Element=Freq
  BusElementIn3 : Inport  Port=7  PortName=VIBus  Element=Id
  BusElementIn4 : Inport  Port=7  PortName=VIBus  Element=Iq
  Constant : Constant  Value=10
  Current_controller : Subsystem
  Inverse Park Transform1 : eeTransforms/Inverse Park Transform  AxisAlignment=Q-axis  PowerInvariant=off
  Reference Current : Subsystem
  Sum2 : Sum  Inputs=|+-
  Terminator : Terminator
  Terminator1 : Terminator
  Unit Delay : UnitDelay  SampleTime=Td
  Unit Delay1 : UnitDelay  SampleTime=Td
  Unit Delay2 : UnitDelay  SampleTime=Ts
  mabc : Outport
  wires:
  QRef/1 -> Reference Current/6(QRef)
  PRef/1 -> Reference Current/5(PRef)
  BusElementIn4/1 -> Current_controller/4(iq)
  BusElementIn3/1 -> Current_controller/2(ipvd)
  BusElementIn1/1 -> Unit Delay1/1
  BusElementIn/1 -> Unit Delay/1
  Unit Delay/1 -> Reference Current/2(V-mag)
  Unit Delay1/1 -> Sum2/2
  Reference Current/1(id_ref) -> Current_controller/1(id-ref)
  Reference Current/2(iq_ref) -> Current_controller/3(iqref)
  Sum2/1 -> Reference Current/3(del f)
  VRef/1 -> Reference Current/1(V_ref)
  FRef/1 -> Sum2/1
  In Bus Element7/1 -> Inverse Park Transform1/2
  In Bus Element3/1 -> Current_controller/5(Vd)
  Current_controller/1(mdq0) -> Inverse Park Transform1/1
  Unit Delay2/1 -> mabc/1
  Inverse Park Transform1/1 -> Unit Delay2/1
  In Bus Element2/1 -> Current_controller/6(Vq)
  Mode/1 -> Terminator/1
  Reset/1 -> Terminator1/1
  Constant/1 -> Reference Current/4(LVRT_iq)
